simulink model "Simulink_5"  (R2013b)
settings: Solver=FixedStepDiscrete  StartTime=0.0  StopTime=1000.0  FixedStep=1  RelTol=1e-3
undefined symbols (not defined in the file): j, magnitude, sigbuilder_block
settings Model: ExtModeAutoUpdateStatusClock=off  Creator=asteele  LastModifiedBy=99900361
settings DataIOCC: SignalLoggingSaveFormat=ModelDataLogs  SignalLoggingName=sigsOut
settings OptimizationCC: BooleanDataType=off
settings DebuggingCC: SaveWithParameterizedLinksMsg=none  SignalResolutionControl=TryResolveAllWithWarning  SolverPrmCheckMsg=none  MultiTaskDSMMsg=warning  MultiTaskCondExecSysMsg=none  StrictBusMsg=None
settings HardwareCC: TargetUnknown=on
settings RTWCC: IncludeERTFirstTime=on
settings GRTTargetCC: CombineOutputUpdateFcns=off  GRTInterface=on

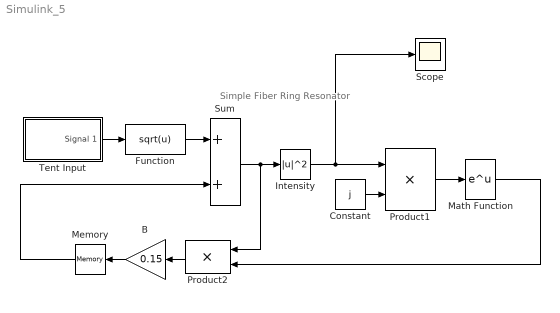
== system Simulink_5 ==
  note: Simple Fiber Ring Resonator
  B : Gain  Gain=0.15  SaturateOnIntegerOverflow=on  OutDataTypeStr=Inherit: Same as input  ParamDataTypeStr=Inherit: Same as input
  Constant : Constant  Value=j
  Function : Fcn  Expr=sqrt(u)
  Intensity : Math  Operator=magnitude^2  SaturateOnIntegerOverflow=on
  Math Function : Math  SaturateOnIntegerOverflow=on
  Memory : Memory
  Product1 : Product  SaturateOnIntegerOverflow=on  InputSameDT=on  OutDataTypeStr=Inherit: Same as first input
  Product2 : Product  SaturateOnIntegerOverflow=on  InputSameDT=on  OutDataTypeStr=Inherit: Same as first input
  Scope : Scope
  Sum : Sum  SaturateOnIntegerOverflow=on  InputSameDT=on  OutDataTypeStr=Inherit: Same as first input
  Tent Input : Subsystem  Tag=STV Subsys  LoadFcn=sigbuilder_block('load');  StartFcn=sigbuilder_block('start');  StopFcn=sigbuilder_block('stop');  ClipboardFcn=sigbuilder_block('clipboard');  mask(Sigbuilder block){}
      mask help: Sigbuilder GUI
      mask init:
      | if ~strcmp(get_param(bdroot(gcb),'SimulationStatus'),'stopped') tuvar = sigbuilder_block('maskInit'); end
      settings: CopyFcn=sigbuilder_block('copy');  DeleteFcn=sigbuilder_block('delete');  ModelCloseFcn=sigbuilder_block('modelClose');  PreSaveFcn=sigbuilder_block('preSave');  NameChangeFcn=sigbuilder_block('namechange');  OpenFcn=sigbuilder_block('open',[50 50 520 400 ]);  CloseFcn=sigbuilder_block('close');
      mask Display: plot(0,0,100,100,[10,10,40,40,10],[80,20,20,80,80],[40,10],[50,50], [40,27,10],[65,72,56],[40,25,25,10],[28,28,43,43]);
  wires:
  Sum/1 -> Intensity/1, Product2/1
  Intensity/1 -> Product1/1, Scope/1
  Product2/1 -> B/1
  B/1 -> Memory/1
  Math Function/1 -> Product2/2
  Constant/1 -> Product1/2
  Product1/1 -> Math Function/1
  Memory/1 -> Sum/2
  Tent Input/1(Signal 1) -> Function/1
  Function/1 -> Sum/1

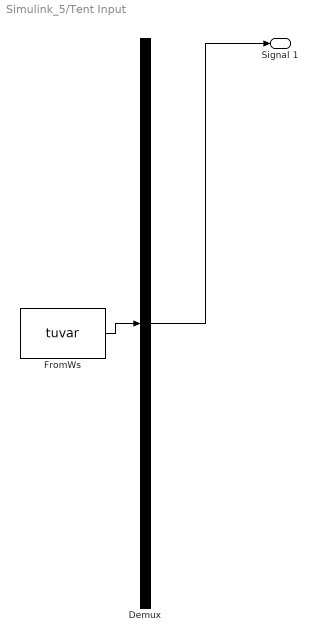
== system Simulink_5/Tent Input ==
  Demux : Demux  Tag=STV Demux  Outputs=1
  FromWs : FromWorkspace  Tag=STV FromWs  VariableName=tuvar  SampleTime=0
      SigBuilderData=|
      | channels.label = 'Signal 1'
      | channels.allXData = {[0 500 1000]}
      | channels.allYData = {[0 9 0]}
      | dataSet.timeRange = [0 1000]
      | dataSet.name = 'Group 1'
  Signal 1 : Outport  Tag=STV Outport
  wires:
  Demux/1 -> Signal 1/1
  FromWs/1 -> Demux/1
